simulink model "FuelPumpTestControl_21a"  (R2021a)
settings: Solver=ode3  StartTime=0.0  StopTime=inf  RelTol=1e-3  EnableMultiTasking=on
values from neighbouring files (symbols this model uses):
  analogReadMax = 1023.0    [SharedData.sldd]
  analogReadMin = 0.0    [SharedData.sldd]
  arduinoSampleTime = 0.01    [SharedData.sldd]
  arduinoVolts = 5.0    [SharedData.sldd]
  batteryCurrentMax = 120.0    [SharedData.sldd]
  batteryCurrentSensorSensitivity = 0.02    [SharedData.sldd]
  batteryVoltageMax = 26.0    [SharedData.sldd]
  batteryVoltageMin = 21.0    [SharedData.sldd]
  batteryVoltReductionFactor = 10.77    [SharedData.sldd]
  controllerFilterCoeff = 3.0    [SharedData.sldd]
  controllerKd = 0.0    [SharedData.sldd]
  controllerKi = 10.0    [SharedData.sldd]
  controllerKp = 0.5    [SharedData.sldd]
  estopMotorSpeed = 0.0    [SharedData.sldd]
  motorCalibrationFactor = 3.0    [SharedData.sldd]
  motorRPMMax = 32000.0    [SharedData.sldd]
  speedCommandMax = 100.0    [SharedData.sldd]
  speedCommandMin = 0.0    [SharedData.sldd]
  stepsBeforeEstop = 4.0    [SharedData.sldd]
undefined symbols (not defined in the file or in its folder): DiscIntNeverNeededParam
libraries: simulink x9, arduinolib x3, dspstat3 x1, arduinosensorlib x1
settings Model: DataDictionary=SharedData.sldd  FPTRunName=Active  SimulationMode=external  EnablePacing=on  ExtModeTrigDuration=2  Creator=Tyler  LastModifiedBy=Tyler
settings SolverCC: AlgebraicLoopSolver=TrustRegion
settings DataIOCC: LimitDataPoints=on  ReturnWorkspaceOutputs=off
settings OptimizationCC: ExpressionDepthLimit=2147483647  LifeSpan=Inf  MaxStackSize=64
settings DebuggingCC: MergeDetectMultiDrivingBlocksExec=none  MultiTaskDSMMsg=none  FcnCallInpInsideContextMsg=warning  BusObjectLabelMismatch=error  AllowSymbolicDim=off  StateNameClashWarn=warning  SFUnexpectedBacktrackingDiag=warning  SFNoUnconditionalDefaultTransitionDiag=warning  SFExecutionAtInitializationDiag=none  ArithmeticOperatorsInVariantConditions=warning
settings HardwareCC: ProdBitPerInt=16  ProdBitPerPointer=16  ProdBitPerSizeT=16  ProdBitPerPtrDiffT=16  ProdLargestAtomicFloat=None  ProdWordSize=8  ProdHWDeviceType=Atmel->AVR
settings ModelReferenceCC: PropagateSignalLabelsOutOfModel=off
settings SFSimCC: SimUseLocalCustomCode=off  CustomCodeUndefinedFunction=UseInterfaceOnly
settings RTWCC: SystemTargetFile=ert.tlc  HardwareBoard=Arduino Uno  TemplateMakefile=ert_default_tmf  RTWVerbose=off  RTWUseLocalCustomCode=off  Toolchain=Arduino AVR  BuildConfiguration=Faster Runs  DLArmComputeVersion=20.02.1
settings CodeAppCC: MangleLength=10  StateflowObjectComments=on
settings ERTTargetCC: MultiwordLength=2048  ERTCustomFileBanners=off  SupportContinuousTime=on  SupportNonInlinedSFcns=on  RemoveResetFunc=off  SupportVariableSizeSignals=on  ModelStepFunctionPrototypeControlCompliant=off  ExtMode=on  ExtModeTransport=3  ExtModeStaticAlloc=on  ExtModeStaticAllocSize=250  ExtModeMexFile=ext_xcp  ExtModeMexArgs=0 4 115200  ExtModeIntrfLevel=Level2 - Open  ConvertIfToSwitch=off  SuppressUnreachableDefaultCases=off
settings ConfigComp: CovMetricSettings=dw  CovSaveCumulativeToWorkspaceVar=on  CovSaveSingleToWorkspaceVar=on  CovExternalEMLEnable=off  CovSFcnEnable=off

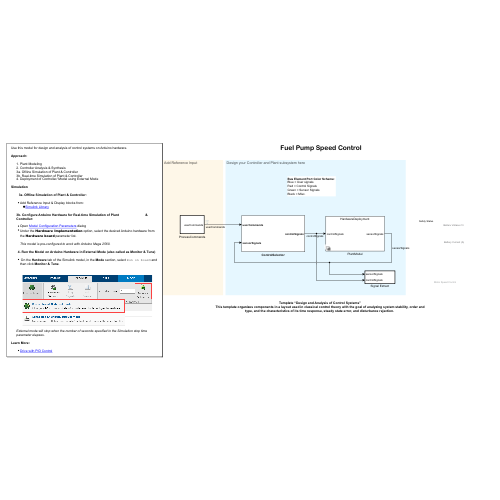
[thumbnail: Simulink's stored preview of the top-level diagram]
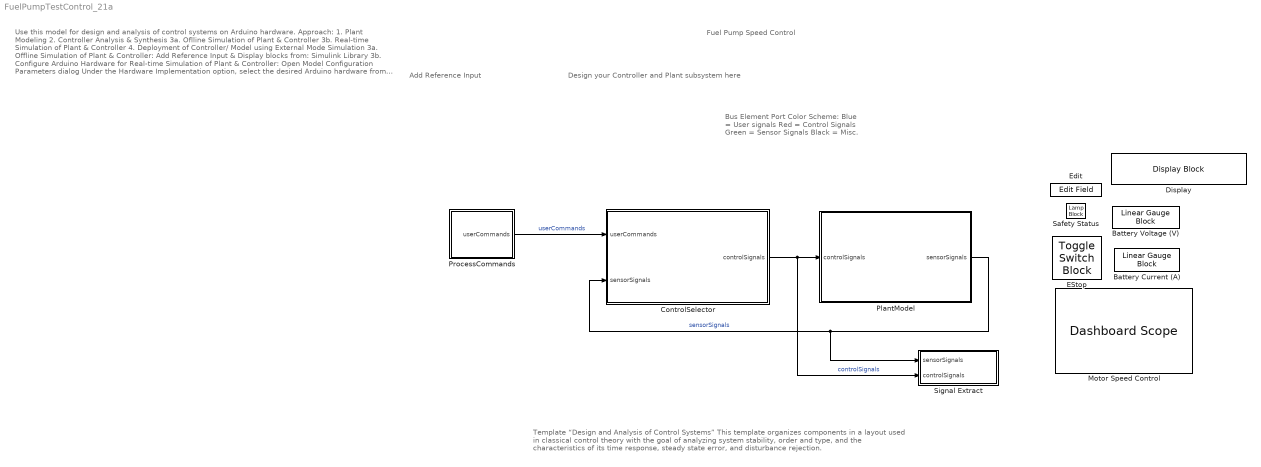
== system FuelPumpTestControl_21a ==
  note: Bus Element Port Color Scheme:
      | Blue = User signals
      | Red = Control Signals
      | Green = Sensor Signals
      | Black = Misc.
  note: Fuel Pump Speed Control
  note: Add Reference Input
  note: Design your Controller and Plant subsystem here
  note: Template “Design and Analysis of Control Systems” This template organizes components in a layout used in classical control theory with the goal of analyzing system stability, order and type, and the characteristics of its time response, steady state error, and disturbance rejection.
  note: Use this model for design and analysis of control systems on Arduino hardware.
      |
      | Approach:
      |
      | 1. Plant Modeling
      | 2. Controller Analysis & Synthesis
      | 3a. Oflline Simulation of Plant & Controller
      | 3b. Real-time Simulation of Plant & Controller
      | 4. Deployment of Controller/ Model using External Mode
      |
      | Simulation
      |
      | 3a. Offline Simulation of Plant & Controller:
      |
      | Add Reference Input & Display blocks from:
      | Simulink Library
      |
      | 3b. Configure Arduino Hardware for Real-time Simulation of Plant & Controller:
      |
      | Open Model Configuration Parameters dialog
      | Under the Hardware Implementation option, select the desired Arduino hardware from the Hardware board parameter list.
      |
      | This model is pre-configured to work with Arduino Mega 2560.
      |
      | 4. Run the Model on Arduino Hardware in External Mode (also called as Monitor & Tune)
      |
      | On the Hardware tab of the Simulink model, in the Mode section, select Run on board and then click Monitor & Tune .
      |
      | External mode will stop when the number of seconds specified in the Simulation stop time parameter elapses.
      |
      | Learn More:
      |
      | Drive with PID Control
  Battery Current (A) : LinearGaugeBlock  LabelPosition=Bottom  ScaleMax=120
  Battery Voltage (V) : LinearGaugeBlock  LabelPosition=Bottom  ScaleMin=20  ScaleMax=26
  ControlSelector : Subsystem  VariantControl=DirectFeed
  Display : DisplayBlock  LabelPosition=Bottom  Transparency=1
  EStop : ToggleSwitchBlock  LabelPosition=Hide
      settings: Values={{'Nominal', 'Emergency Stop'}, [0 1]}
  Edit : EditField  LabelPosition=Hide  ShowInitialText=on  Alignment=Center
  Motor Speed Control : DashboardScope  Ymin=0  Ymax=100  ScaleAtStop=off  UpdateMode=Scroll
  PlantModel : Subsystem  Variant=on  VariantControlMode=label  VariantControl=plantModel==1  LabelModeActiveChoice=HardwareDeployment
  ProcessCommands : Subsystem  TreatAsAtomicUnit=on
  Safety Status : LampBlock  LabelPosition=Hide
  Signal Extract : Subsystem  TreatAsAtomicUnit=on
  wires:
  PlantModel/1(sensorSignals) -> Signal Extract/1(sensorSignals), ControlSelector/2(sensorSignals)  "sensorSignals"
  ControlSelector/1(controlSignals) -> Signal Extract/2(controlSignals), PlantModel/1(controlSignals)  "controlSignals"
  ProcessCommands/1(userCommands) -> ControlSelector/1(userCommands)  "userCommands"

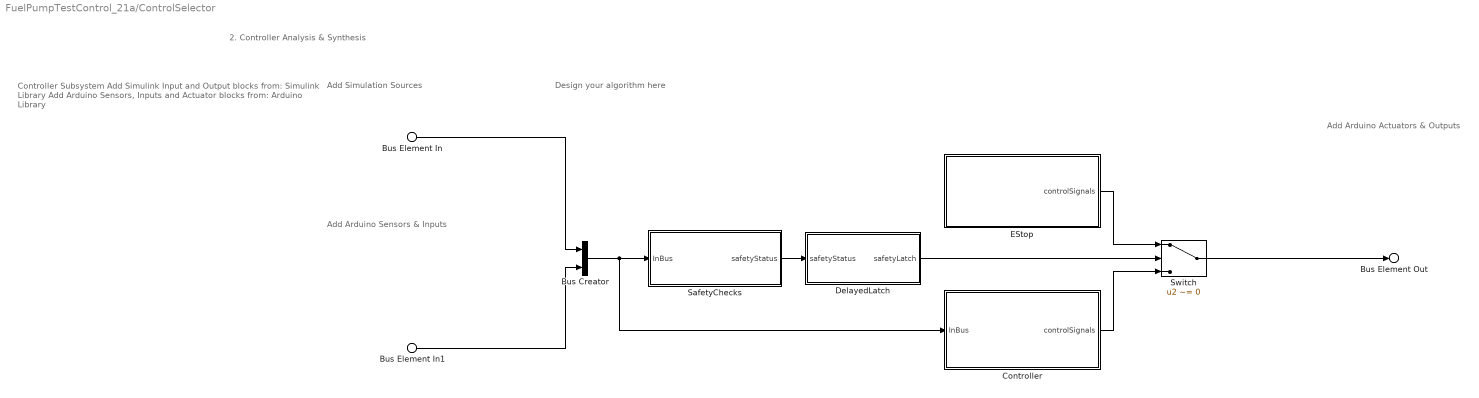
== system FuelPumpTestControl_21a/ControlSelector ==
  note: 2. Controller Analysis & Synthesis
  note: Add Arduino Sensors & Inputs
  note: Design your algorithm here
  note: Add Simulation Sources
  note: Add Arduino Actuators & Outputs
  note: Controller Subsystem
      |
      | Add Simulink Input and Output blocks from:
      | Simulink Library
      | Add Arduino Sensors, Inputs and Actuator blocks from:
      | Arduino Library
  Bus Element In : Inport  PortName=userCommands
  Bus Element In1 : Inport  Port=2  PortName=sensorSignals
  Bus Creator : BusCreator  Inputs=2
  Controller : Subsystem  TreatAsAtomicUnit=on  Variant=on  VariantControlMode=label  LabelModeActiveChoice=PID
  DelayedLatch : Subsystem  TreatAsAtomicUnit=on
  EStop : Subsystem  TreatAsAtomicUnit=on
  SafetyChecks : Subsystem  TreatAsAtomicUnit=on
  Switch : Switch  Criteria=u2 ~= 0
  Bus Element Out : Outport  PortName=controlSignals
  wires:
  Bus Element In1/1 -> Bus Creator/2
  Bus Element In/1 -> Bus Creator/1
  Bus Creator/1 -> Controller/1(InBus), SafetyChecks/1(InBus)
  Switch/1 -> Bus Element Out/1
  SafetyChecks/1(safetyStatus) -> DelayedLatch/1(safetyStatus)
  DelayedLatch/1(safetyLatch) -> Switch/2
  Controller/1(controlSignals) -> Switch/3
  EStop/1(controlSignals) -> Switch/1

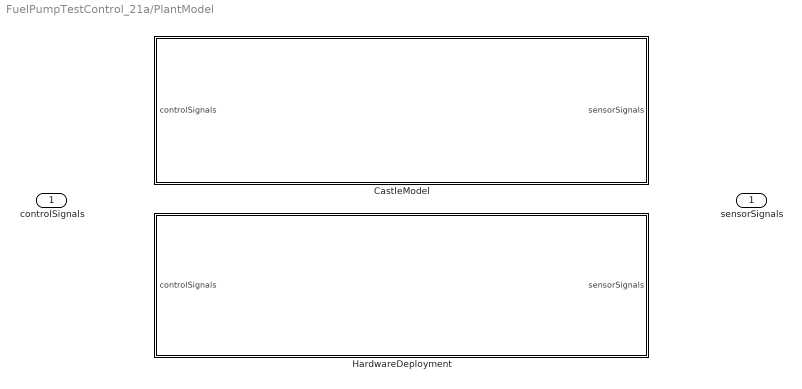
== system FuelPumpTestControl_21a/PlantModel ==
  controlSignals : Inport
  CastleModel : Subsystem  VariantControl=CastleModel
  HardwareDeployment : Subsystem  VariantControl=HardwareDeployment
  sensorSignals : Outport

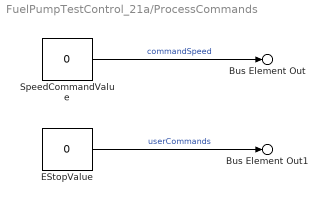
== system FuelPumpTestControl_21a/ProcessCommands ==
  EStopValue : Constant  Value=0  OutMin=0  OutMax=100  OutDataTypeStr=double
  SpeedCommandValue : Constant  Value=0  OutMin=0  OutMax=100  OutDataTypeStr=double
  Bus Element Out : Outport  PortName=userCommands  Element=motorSpeed
  Bus Element Out1 : Outport  PortName=userCommands  Element=estop
  wires:
  SpeedCommandValue/1 -> Bus Element Out/1  "commandSpeed"
  EStopValue/1 -> Bus Element Out1/1  "userCommands"

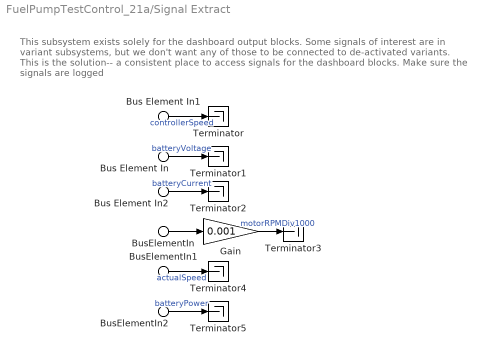
== system FuelPumpTestControl_21a/Signal Extract ==
  note: This subsystem exists solely for the dashboard output blocks. Some signals of interest are in variant subsystems, but we don't want any of those to be connected to de-activated variants. This is the solution-- a consistent place to access signals for the dashboard blocks. Make sure the signals are logged
  Bus Element In : Inport  PortName=sensorSignals  Element=batteryVoltage
  Bus Element In2 : Inport  PortName=sensorSignals  Element=batteryCurrent
  BusElementIn : Inport  PortName=sensorSignals  Element=motorSpeed
  BusElementIn1 : Inport  PortName=sensorSignals  Element=motorSpeedScaled
  BusElementIn2 : Inport  PortName=sensorSignals  Element=batteryPower
  Bus Element In1 : Inport  Port=2  PortName=controlSignals  Element=motorSpeed
  Gain : Gain  Gain=0.001
  Terminator{,1..5} (6 alike) : Terminator
  wires:
  Bus Element In1/1 -> Terminator/1  "controllerSpeed"
  Bus Element In/1 -> Terminator1/1  "batteryVoltage"
  BusElementIn/1 -> Gain/1
  Bus Element In2/1 -> Terminator2/1  "batteryCurrent"
  BusElementIn1/1 -> Terminator4/1  "actualSpeed"
  BusElementIn2/1 -> Terminator5/1  "batteryPower"
  Gain/1 -> Terminator3/1  "motorRPMDiv1000"

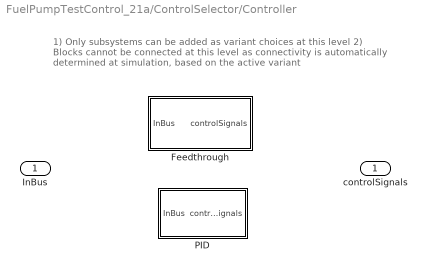
== system FuelPumpTestControl_21a/ControlSelector/Controller ==
  note: 1) Only subsystems can be added as variant choices at this level
      | 2) Blocks cannot be connected at this level as connectivity is
      | automatically determined at simulation, based on the active variant
  InBus : Inport
  Feedthrough : Subsystem  VariantControl=Feedthrough
  PID : Subsystem  TreatAsAtomicUnit=on  VariantControl=PID
  controlSignals : Outport  VectorParamsAs1DForOutWhenUnconnected=off

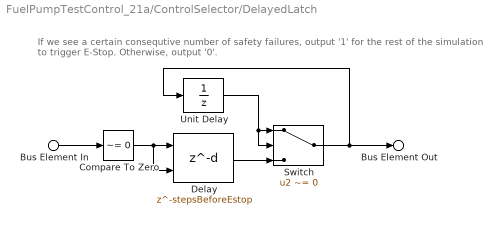
== system FuelPumpTestControl_21a/ControlSelector/DelayedLatch ==
  note: If we see a certain consequtive number of safety failures, output '1' for the rest of the simulation to trigger E-Stop. Otherwise, output '0'.
  Bus Element In : Inport  PortName=safetyStatus
  Compare To Zero : simulink/Logic and Bit Operations/Compare To Zero  relop=~=  OutDataTypeStr=boolean
  Delay : Delay  DelayLength=stepsBeforeEstop  ExternalReset=Falling
      settings: InputPortMap=u0,r5
  Switch : Switch  Criteria=u2 ~= 0
  Unit Delay : UnitDelay  SampleTime=-1  HasFrameUpgradeWarning=on
  Bus Element Out : Outport  PortName=safetyLatch
  wires:
  Unit Delay/1 -> Switch/2, Switch/1
  Switch/1 -> Bus Element Out/1, Unit Delay/1
  Delay/1 -> Switch/3
  Bus Element In/1 -> Compare To Zero/1
  Compare To Zero/1 -> Delay/2, Delay/1

== system FuelPumpTestControl_21a/ControlSelector/EStop ==
  EstopMotor : Constant  Value=estopMotorSpeed  OutDataTypeStr=Inherit: Inherit via back propagation
  Bus Element Out1 : Outport  PortName=controlSignals  Element=motorSpeed
  wires:
  EstopMotor/1 -> Bus Element Out1/1

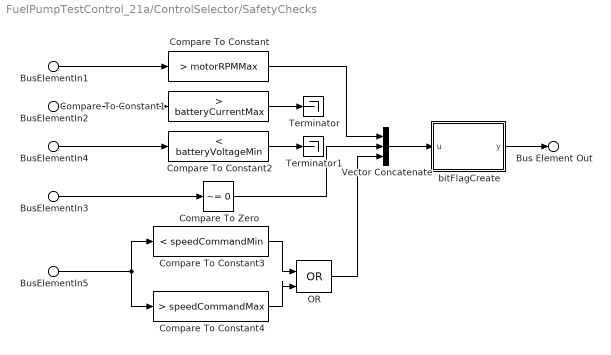
== system FuelPumpTestControl_21a/ControlSelector/SafetyChecks ==
  BusElementIn1 : Inport  PortName=InBus  Element=sensorSignals.motorSpeed
  BusElementIn2 : Inport  PortName=InBus  Element=sensorSignals.batteryCurrent
  BusElementIn4 : Inport  PortName=InBus  Element=sensorSignals.batteryVoltage
  BusElementIn5 : Inport  PortName=InBus  Element=userCommands.motorSpeed
  BusElementIn3 : Inport  PortName=InBus  Element=userCommands.estop
  Compare To Constant : simulink/Logic and Bit Operations/Compare To Constant  relop=>  const=motorRPMMax  OutDataTypeStr=boolean
  Compare To Constant1 : simulink/Logic and Bit Operations/Compare To Constant  relop=>  const=batteryCurrentMax  OutDataTypeStr=boolean
  Compare To Constant2 : simulink/Logic and Bit Operations/Compare To Constant  relop=<  const=batteryVoltageMin  OutDataTypeStr=boolean
  Compare To Constant3 : simulink/Logic and Bit Operations/Compare To Constant  relop=<  const=speedCommandMin  OutDataTypeStr=boolean
  Compare To Constant4 : simulink/Logic and Bit Operations/Compare To Constant  relop=>  const=speedCommandMax  OutDataTypeStr=boolean
  Compare To Zero : simulink/Logic and Bit Operations/Compare To Zero  relop=~=  OutDataTypeStr=boolean
  OR : Logic  Operator=OR  IconShape=distinctive  AllPortsSameDT=off  OutDataTypeStr=boolean
  Terminator : Terminator
  Terminator1 : Terminator
  Vector Concatenate : Concatenate  NumInputs=3
  bitFlagCreate : MATLAB Function  TreatAsAtomicUnit=on
  Bus Element Out : Outport  PortName=safetyStatus
  wires:
  BusElementIn4/1 -> Compare To Constant2/1
  Compare To Constant3/1 -> OR/1
  BusElementIn2/1 -> Compare To Constant1/1
  Vector Concatenate/1 -> bitFlagCreate/1(u)
  BusElementIn5/1 -> Compare To Constant3/1, Compare To Constant4/1
  BusElementIn1/1 -> Compare To Constant/1
  Compare To Constant/1 -> Vector Concatenate/1
  Compare To Constant4/1 -> OR/2
  bitFlagCreate/1(y) -> Bus Element Out/1
  BusElementIn3/1 -> Compare To Zero/1
  Compare To Zero/1 -> Vector Concatenate/2
  OR/1 -> Vector Concatenate/3
  Compare To Constant1/1 -> Terminator/1
  Compare To Constant2/1 -> Terminator1/1

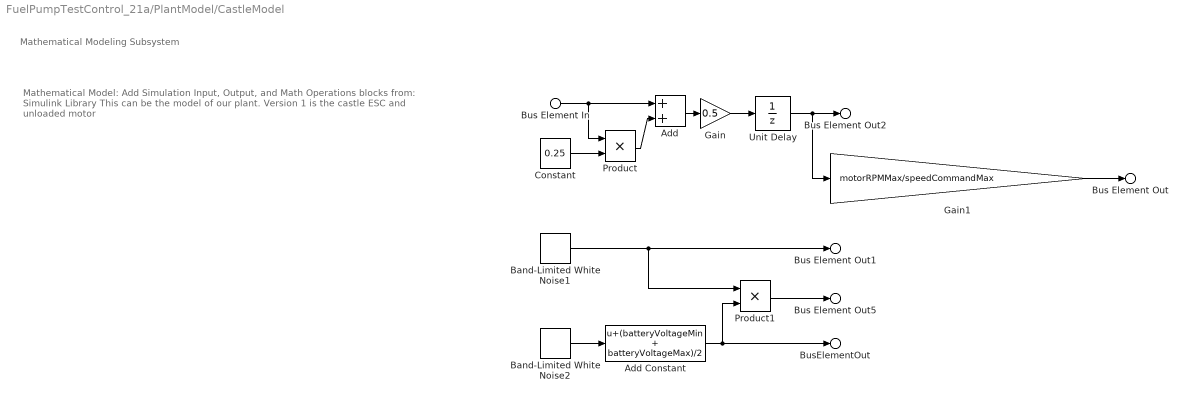
== system FuelPumpTestControl_21a/PlantModel/CastleModel ==
  note: Mathematical Model:
      |
      | Add Simulation Input, Output, and Math Operations blocks from:
      | Simulink Library
      | This can be the model of our plant. Version 1 is the castle ESC and unloaded motor
  note: Mathematical Modeling Subsystem
  Bus Element In : Inport  PortName=controlSignals  Element=motorSpeed
  Add : Sum
  Add Constant : Bias  Bias=(batteryVoltageMin + batteryVoltageMax)/2
  Band-Limited White Noise1 : simulink/Sources/Band-Limited White Noise  Cov=[0.1]  Ts=0.1  seed=[1597]
  Band-Limited White Noise2 : simulink/Sources/Band-Limited White Noise  Cov=[0.1]  Ts=0.1  seed=[23341]
  Constant : Constant  Value=0.25  SampleTime=-1
  Gain : Gain  Gain=0.5
  Gain1 : Gain  Gain=motorRPMMax/speedCommandMax
  Product : Product
  Product1 : Product
  Unit Delay : UnitDelay  SampleTime=-1  HasFrameUpgradeWarning=on
  Bus Element Out1 : Outport  PortName=sensorSignals  Element=batteryCurrent
  BusElementOut : Outport  PortName=sensorSignals  Element=batteryVoltage
  Bus Element Out2 : Outport  PortName=sensorSignals  Element=motorSpeedScaled
  Bus Element Out : Outport  PortName=sensorSignals  Element=motorSpeed
  Bus Element Out5 : Outport  PortName=sensorSignals  Element=batteryPower
  wires:
  Bus Element In/1 -> Product/1, Add/1
  Add/1 -> Gain/1
  Product/1 -> Add/2
  Gain/1 -> Unit Delay/1
  Constant/1 -> Product/2
  Unit Delay/1 -> Gain1/1, Bus Element Out2/1
  Band-Limited White Noise1/1 -> Product1/1, Bus Element Out1/1
  Band-Limited White Noise2/1 -> Add Constant/1
  Add Constant/1 -> BusElementOut/1, Product1/2
  Product1/1 -> Bus Element Out5/1
  Gain1/1 -> Bus Element Out/1

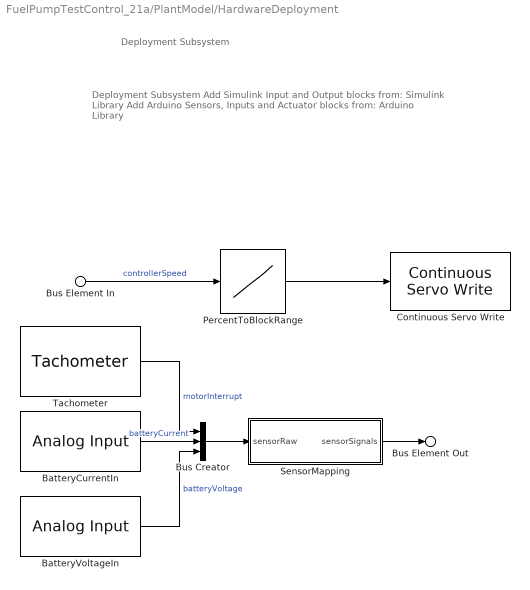
== system FuelPumpTestControl_21a/PlantModel/HardwareDeployment ==
  note: Deployment Subsystem
  note: Deployment Subsystem
      | Add Simulink Input and Output blocks from:
      | Simulink Library
      | Add Arduino Sensors, Inputs and Actuator blocks from:
      | Arduino Library
  Bus Element In : Inport  PortName=controlSignals  Element=motorSpeed
  BatteryCurrentIn : arduinolib/Analog Input  pinNumber=arduinoCurrentPin  ReadResultsOnly=off  ConversionTriggerSource=Software  ExternalTriggerType=uint32(0)  OutputDataType=uint16  EnableConversionCompleteNotify=off  EnableOuputStatus=off  SampleTime=arduinoSampleTime  blockPlatform=arduino
  BatteryVoltageIn : arduinolib/Analog Input  pinNumber=arduinoBattVoltagePin  ReadResultsOnly=off  ConversionTriggerSource=Software  ExternalTriggerType=uint32(0)  OutputDataType=uint16  EnableConversionCompleteNotify=off  EnableOuputStatus=off  SampleTime=arduinoSampleTime  blockPlatform=arduino
  Bus Creator : BusCreator  Inputs=3
  Continuous Servo Write : arduinolib/Continuous Servo Write  pinNumber=arduinoPWMPin  ServoIndex=0  blockPlatform=ARDUINO
  PercentToBlockRange : Lookup_n-D  NumberOfTableDimensions=1  BreakpointsForDimension1=[speedCommandMin speedCommandMax]  Table=[0 90]  InternalRulePriority=Speed  RndMeth=Simplest  InputSameDT=on
  SensorMapping : Subsystem
  Tachometer : arduinosensorlib/Tachometer  PinNumber=2  InterruptMode=RISING  PulseCountperRotation=1  SampleTime=arduinoSampleTime  blockPlatform=ARDUINO
  Bus Element Out : Outport  PortName=sensorSignals
  wires:
  BatteryCurrentIn/1 -> Bus Creator/2  "batteryCurrent"
  BatteryVoltageIn/1 -> Bus Creator/3  "batteryVoltage"
  SensorMapping/1(sensorSignals) -> Bus Element Out/1
  Tachometer/1 -> Bus Creator/1  "motorInterrupt"
  Bus Creator/1 -> SensorMapping/1(sensorRaw)
  Bus Element In/1 -> PercentToBlockRange/1  "controllerSpeed"
  PercentToBlockRange/1 -> Continuous Servo Write/1

== system FuelPumpTestControl_21a/ControlSelector/Controller/Feedthrough ==
  Bus Element In : Inport  PortName=InBus  Element=userCommands.motorSpeed
  Bus Element Out : Outport  PortName=controlSignals  Element=motorSpeed
  wires:
  Bus Element In/1 -> Bus Element Out/1

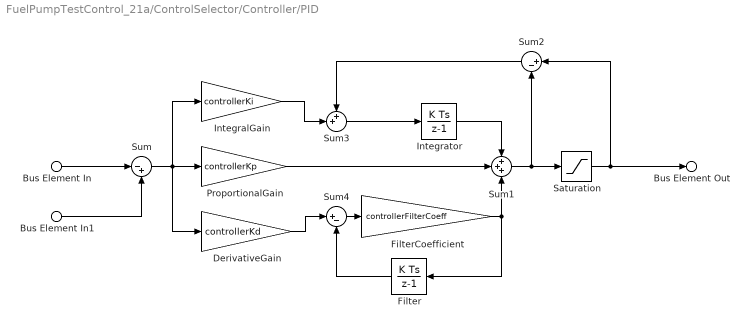
== system FuelPumpTestControl_21a/ControlSelector/Controller/PID ==
  Bus Element In1 : Inport  PortName=InBus  Element=userCommands.motorSpeed
  Bus Element In : Inport  PortName=InBus  Element=sensorSignals.motorSpeedScaled
  DerivativeGain : Gain  Gain=controllerKd
  Filter : DiscreteIntegrator  SampleTime=-1  ICPrevOutput=DiscIntNeverNeededParam  ICPrevScaledInput=DiscIntNeverNeededParam
  FilterCoefficient : Gain  Gain=controllerFilterCoeff
  IntegralGain : Gain  Gain=controllerKi
  Integrator : DiscreteIntegrator  SampleTime=-1  ICPrevOutput=DiscIntNeverNeededParam  ICPrevScaledInput=DiscIntNeverNeededParam
  ProportionalGain : Gain  Gain=controllerKp
  Saturation : Saturate  UpperLimit=speedCommandMax  LowerLimit=speedCommandMin
      settings: AttributesFormatString=%<LowerLimit> to %<UpperLimit>
  Sum : Sum  Inputs=|-+
  Sum1 : Sum  Inputs=+++
  Sum2 : Sum  Inputs=|+-
  Sum3 : Sum  Inputs=++|
  Sum4 : Sum  Inputs=|+-
  Bus Element Out : Outport  PortName=controlSignals  Element=motorSpeed
  wires:
  Bus Element In1/1 -> Sum/2
  IntegralGain/1 -> Sum3/2
  Sum3/1 -> Integrator/1
  DerivativeGain/1 -> Sum4/1
  Sum4/1 -> FilterCoefficient/1
  Sum2/1 -> Sum3/1
  Sum1/1 -> Saturation/1, Sum2/2
  Filter/1 -> Sum4/2
  Sum/1 -> DerivativeGain/1, ProportionalGain/1, IntegralGain/1
  Integrator/1 -> Sum1/1
  ProportionalGain/1 -> Sum1/2
  FilterCoefficient/1 -> Sum1/3, Filter/1
  Bus Element In/1 -> Sum/1
  Saturation/1 -> Bus Element Out/1, Sum2/1

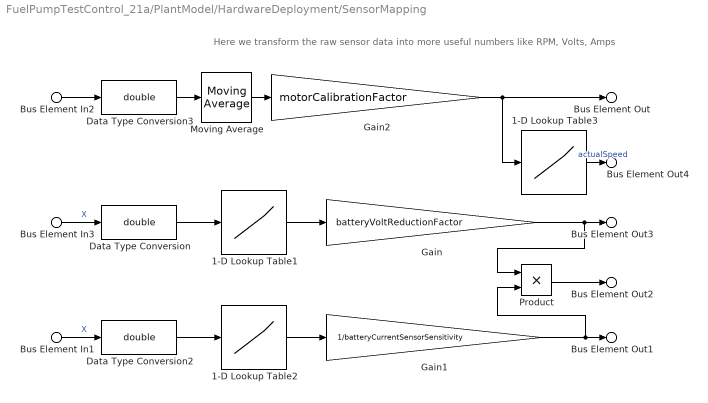
== system FuelPumpTestControl_21a/PlantModel/HardwareDeployment/SensorMapping ==
  note: Here we transform the raw sensor data into more useful numbers like RPM, Volts, Amps
  Bus Element In3 : Inport  PortName=sensorRaw  Element=batteryVoltage
  Bus Element In1 : Inport  PortName=sensorRaw  Element=batteryCurrent
  Bus Element In2 : Inport  PortName=sensorRaw  Element=motorInterrupt
  1-D Lookup Table1 : Lookup_n-D  NumberOfTableDimensions=1  BreakpointsForDimension1=[analogReadMin analogReadMax]  Table=[0 arduinoVolts]  InternalRulePriority=Speed  RndMeth=Simplest  InputSameDT=on
  1-D Lookup Table2 : Lookup_n-D  NumberOfTableDimensions=1  BreakpointsForDimension1=[analogReadMin analogReadMax]  Table=[0 arduinoVolts]  InternalRulePriority=Speed  RndMeth=Simplest  InputSameDT=on
  1-D Lookup Table3 : Lookup_n-D  NumberOfTableDimensions=1  BreakpointsForDimension1=[0 motorRPMMax]  Table=[speedCommandMin speedCommandMax]  InternalRulePriority=Speed  RndMeth=Simplest  InputSameDT=on
  Data Type Conversion : DataTypeConversion  OutDataTypeStr=double
  Data Type Conversion2 : DataTypeConversion  OutDataTypeStr=double
  Data Type Conversion3 : DataTypeConversion  OutDataTypeStr=double
  Gain : Gain  Gain=batteryVoltReductionFactor
  Gain1 : Gain  Gain=1/batteryCurrentSensorSensitivity
  Gain2 : Gain  Gain=motorCalibrationFactor
  Moving Average : dspstat3/Moving Average  Method=Sliding window  ForgettingFactorPort=off  SpecifyWindowLength=on  WindowLength=30  ForgettingFactor=0.9  SimulateUsing=Code generation
  Product : Product
  Bus Element Out : Outport  PortName=sensorSignals  Element=motorSpeed
  Bus Element Out3 : Outport  PortName=sensorSignals  Element=batteryVoltage
  Bus Element Out1 : Outport  PortName=sensorSignals  Element=batteryCurrent
  Bus Element Out2 : Outport  PortName=sensorSignals  Element=batteryPower
  Bus Element Out4 : Outport  PortName=sensorSignals  Element=motorSpeedScaled
  wires:
  Bus Element In1/1 -> Data Type Conversion2/1  "X"
  Bus Element In3/1 -> Data Type Conversion/1  "X"
  Data Type Conversion/1 -> 1-D Lookup Table1/1
  Data Type Conversion2/1 -> 1-D Lookup Table2/1
  Gain/1 -> Product/1, Bus Element Out3/1
  Gain1/1 -> Product/2, Bus Element Out1/1
  Product/1 -> Bus Element Out2/1
  1-D Lookup Table2/1 -> Gain1/1
  1-D Lookup Table1/1 -> Gain/1
  1-D Lookup Table3/1 -> Bus Element Out4/1  "actualSpeed"
  Bus Element In2/1 -> Data Type Conversion3/1
  Data Type Conversion3/1 -> Moving Average/1
  Gain2/1 -> Bus Element Out/1, 1-D Lookup Table3/1
  Moving Average/1 -> Gain2/1

== matlab function FuelPumpTestControl_21a/ControlSelector/SafetyChecks/bitFlagCreate ==
  data: u input; y output
function y = bitFlagCreate(u)
y = uint8(0);
for n = 1:length(u)
    y = y + 2^(n-1) * u(n);
end
y = uint8(0);
